simulink model "task1"  (R2024a)
settings: Solver=VariableStepAuto  StartTime=0.0  StopTime=10.0  MaxStep=0.01  RelTol=1e-3
undefined symbols (not defined in the file): A, B, Bf, C, D, Df, Gamma_f, Gamma_g, K, Kf, Kg, wf0, wg0, x0, Yf, Yg
settings Model: Creator=sizgr  LastModifiedBy=sizgr

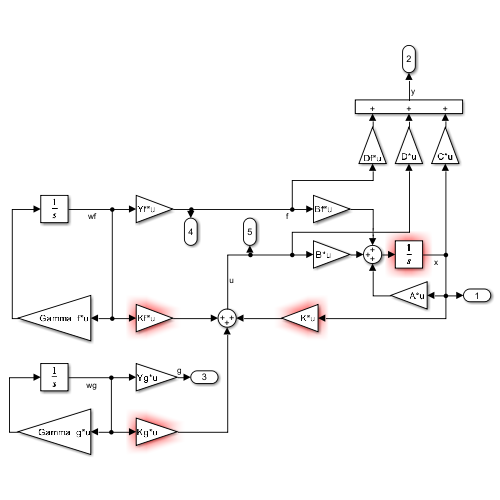
[thumbnail: Simulink's stored preview of the top-level diagram]
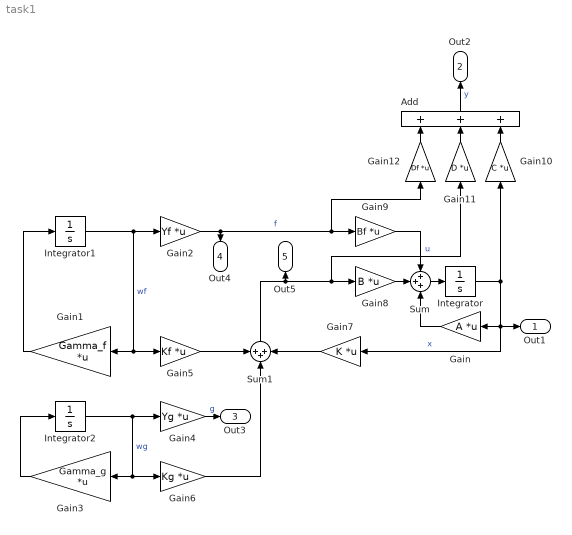
== system task1 ==
  Add : Sum  Inputs=+++
  Gain : Gain  Gain=A  Multiplication=Matrix(K*u)
  Gain1 : Gain  Gain=Gamma_f  Multiplication=Matrix(K*u)
  Gain10 : Gain  Gain=C  Multiplication=Matrix(K*u)
  Gain11 : Gain  Gain=D  Multiplication=Matrix(K*u)
  Gain12 : Gain  Gain=Df  Multiplication=Matrix(K*u)
  Gain2 : Gain  Gain=Yf  Multiplication=Matrix(K*u)
  Gain3 : Gain  Gain=Gamma_g  Multiplication=Matrix(K*u)
  Gain4 : Gain  Gain=Yg  Multiplication=Matrix(K*u)
  Gain5 : Gain  Gain=Kf  Multiplication=Matrix(K*u)
  Gain6 : Gain  Gain=Kg  Multiplication=Matrix(K*u)
  Gain7 : Gain  Gain=K  Multiplication=Matrix(K*u)
  Gain8 : Gain  Gain=B  Multiplication=Matrix(K*u)
  Gain9 : Gain  Gain=Bf  Multiplication=Matrix(K*u)
  Integrator : Integrator  InitialCondition=x0
  Integrator1 : Integrator  InitialCondition=wf0
  Integrator2 : Integrator  InitialCondition=wg0
  Sum : Sum  Inputs=+++
  Sum1 : Sum  Inputs=+++
  Out1 : Outport
  Out2 : Outport  Port=2
  Out3 : Outport  Port=3
  Out4 : Outport  Port=4
  Out5 : Outport  Port=5
  wires:
  Sum/1 -> Integrator/1
  Gain/1 -> Sum/3
  Integrator/1 -> Gain/1, Gain7/1, Out1/1, Gain10/1  "x"
  Integrator1/1 -> Gain2/1, Gain1/1, Gain5/1  "wf"
  Gain1/1 -> Integrator1/1
  Gain3/1 -> Integrator2/1
  Integrator2/1 -> Gain4/1, Gain3/1, Gain6/1  "wg"
  Gain5/1 -> Sum1/1
  Gain6/1 -> Sum1/2
  Gain7/1 -> Sum1/3
  Gain8/1 -> Sum/2
  Gain9/1 -> Sum/1
  Sum1/1 -> Gain11/1, Gain8/1, Out5/1  "u"
  Gain2/1 -> Gain12/1, Gain9/1, Out4/1  "f"
  Gain10/1 -> Add/3
  Gain11/1 -> Add/2
  Gain12/1 -> Add/1
  Add/1 -> Out2/1  "y"
  Gain4/1 -> Out3/1  "g"
